simulink model "manualInputSim"  (R2025b)
settings: Solver=VariableStepAuto  StartTime=0.0  StopTime=inf  RelTol=1e-3
undefined symbols (not defined in the file or in its folder): SteerLim, VEH
libraries: sim3dlib x7, sim3dautolib x2, simulink_extras x1, vehicle_sim_lib x1
(part 1 of 2)
settings Model: Creator=bigch  LastModifiedBy=bigch

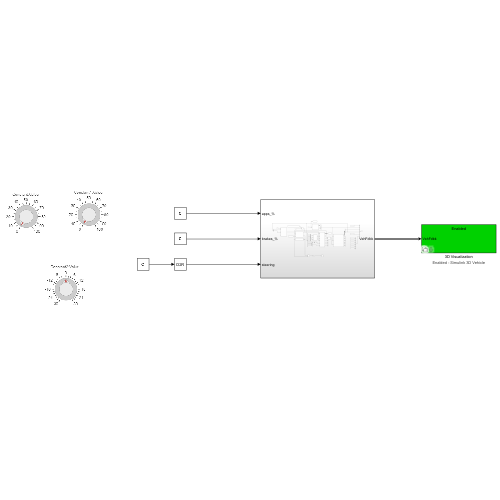
[thumbnail: Simulink's stored preview of the top-level diagram]
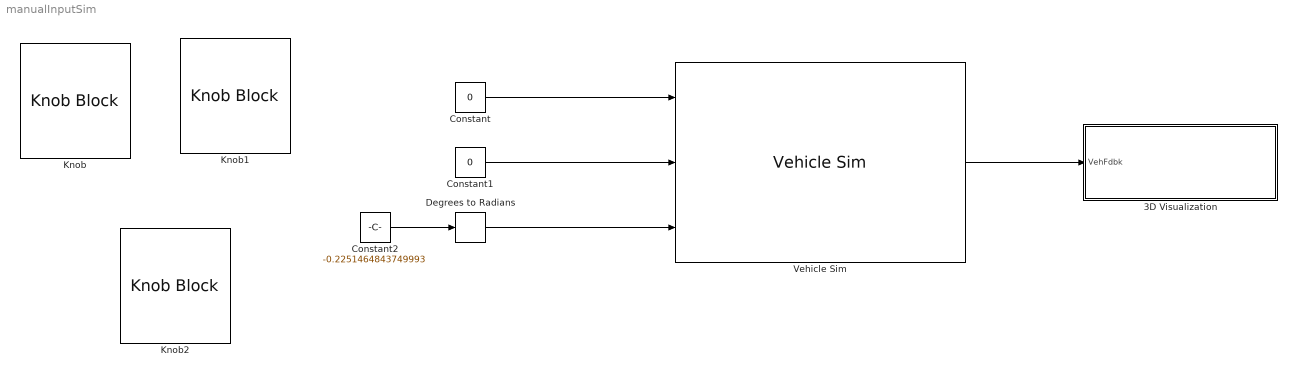
== system manualInputSim ==
  3D Visualization : Subsystem  Variant=on  VariantControl=Choice  mask(3D Visualization Setup){engine3D=Enabled - Simulink 3D Vehicle, conesOn=off, annotOn=off, pathOn=off, InitialPos=[ 0, 0, 0 ], InitialRot=[0, 0, 0], Ts=1/60}
      mask prompts: engine3D "Visualization Mode:"; conesOn "Include cones"; annotOn "Include annotations"; pathOn "Include path markers"; InitialPos "shared_sim3dblks:sim3dblkVehicleWithGroundFollowingVDBS:blkPrm_InitialPos"; InitialRot "shared_sim3dblks:sim3dblkVehicleWithGroundFollowingVDBS:blkPrm_InitialRotSAE"; Ts "shared_sim3dblks:sim3dblkConfig:Ts"
      mask help: This is an example specific block designed to only work with vydnblksskidpad.slx. It is used in conjuction with the vehicle subystem to provide options for the 3D game engine visualization (requires Simulink 3D Animation).
      mask init:
      | visType = get_param(gcb,"engine3D");
      | switch visType
      |     case "Disabled"
      |         autoblksenableparameters(gcb, [],{'conesOn';'annotOn';'pathOn'},[],[],true);
      |         set_param([bdroot '/Formula Student Vehicle'],'vehType','Simulink Physics')
      |     case "Enabled - Ground Following Vehicle"
      |         set_param([bdroot '/Formula Student Vehicle'],'vehType','Simulink Physics')
      |         autoblksenableparameters(gcb, {'conesOn';'annotOn';'pathOn'},[],[],[],true);
      |     case "Enabled - Game Physics Vehicle"
      |         set_param([bdroot '/Formula Student Vehicle'],'vehType','Game Engine Physics')
      |         autoblksenableparameters(gcb, {'conesOn';'annotOn';'pathOn'},[],[],[],true);
      | end
      settings: AttributesFormatString=%<engine3D>
      mask TypeOptions engine3D: Disabled | Enabled - Simulink 3D Vehicle | Enabled - Game Physics Vehicle
      mask Callback engine3D:
      | if strcmp(get_param(gcb,"engine3D"),"Disabled")
      |     autoblksenableparameters(gcb, [],{'conesOn';'annotOn';'pathOn'},[],[],true);
      | else
      |     autoblksenableparameters(gcb, {'conesOn';'annotOn';'pathOn'},[],[],[],true);
      | end
      mask DialogControl InitialPos Prompt: Initial position [X, Y, Z], InitialPos [m]:
      mask DialogControl InitialRot Prompt: Initial rotation [Roll, Pitch, Yaw], InitialRot [rad]:
      mask DialogControl Ts Prompt: Sample time:
  Constant : Constant  Value=0
  Constant1 : Constant  Value=0
  Constant2 : Constant  Value=-0.2251464843749993
  Degrees to Radians : simulink_extras/Transformations/Degrees to Radians
  Knob : KnobBlock
  Knob1 : KnobBlock
  Knob2 : KnobBlock  ScaleMin=-30  ScaleMax=30
  Vehicle Sim : vehicle_sim_lib/Vehicle Sim  SystemSampleTime=-1  VariantActivationTime=update diagram  EmptyChoice=off  PassThrough=off  PassThroughVariantControl=(default)  EmptyChoiceVariantControl=(default)  AllowFlexibleInterface=on  Latency=0  AutoFrameSizeCalculation=off
  wires:
  Constant1/1 -> Vehicle Sim/2
  Degrees to Radians/1 -> Vehicle Sim/3
  Vehicle Sim/1 -> 3D Visualization/1(VehFdbk)
  Constant/1 -> Vehicle Sim/1
  Constant2/1 -> Degrees to Radians/1

== system manualInputSim/3D Visualization ==
  VehFdbk : Inport
  Disabled : Subsystem  VariantControl=engine3D==1
  Enabled : Subsystem  VariantControl=engine3D~=1

== system manualInputSim/3D Visualization/Disabled ==

== system manualInputSim/3D Visualization/Enabled ==
  VehFdbk : Inport
  3D Visualization : Subsystem  Variant=on  VariantControl=Choice
  Cones : Subsystem  Variant=on  VariantControl=Choice
  wires:
  VehFdbk/1 -> 3D Visualization/1(VehFdbk)

== system manualInputSim/3D Visualization/Enabled/3D Visualization ==
  VehFdbk : Inport
  Disabled : Subsystem  VariantControl=engine3D==1
  Ground Following : Subsystem  VariantControl=engine3D==4
  Physical Vehicle : Subsystem  VariantControl=engine3D==3
  Simulation 3D Vehicle : Subsystem  VariantControl=engine3D==2

== system manualInputSim/3D Visualization/Enabled/Cones ==
  Disabled : Subsystem  VariantControl=conesOn==0
  Enabled : Subsystem  VariantControl=conesOn==1

== system manualInputSim/3D Visualization/Enabled/3D Visualization/Disabled ==

== system manualInputSim/3D Visualization/Enabled/3D Visualization/Ground Following ==
  VehFdbk : Inport
  Annotations : Subsystem  Variant=on  VariantControl=Annotations
  Bus Selector3 : BusSelector  OutputSignals=VehFdbk.InertFrm.Cg.Disp.X,VehFdbk.InertFrm.Cg.Disp.Y,VehFdbk.InertFrm.Cg.Ang.psi,Driver.Light controls
  Path : Subsystem  Variant=on  VariantControl=Choice
  Simulation 3D Scene Configuration : sim3dlib/Simulation 3D Scene Configuration  Priority=0  ProjectFormat=Default Scenes  SceneDesc=Open surface  ProjectName=C:\Program Files\MATLAB\R2025b\toolbox\shared\sim3d_projects\automotive_project_windows\UE\WindowsNoEditor\VehicleSimulation.exe  ScenePath=/Game/Maps/HwStrght  EnableOpenDRIVE=off  vehTagList={'Custom';'GamePhysVehPath';'GrndVehPath';'Scene Origin';'Sim3dActor1';'SimulinkPhysVehPath';'SimulinkVehicle1';'SimulinkVehicle2';'SimulinkVehicle3'}  vehTag=SimulinkVehicle3  AttachedCameraRelativeTranslation=[0 0 0]  FreeCameraDefaultInitialTranslation=[-6, 0, 2]  AttachedCameraRelativeRotation=[0 0 0]  FreeCameraDefaultInitialRotation=[0, -15, 0]  ViewpointName=Custom  FreeCameraInitialTranslation=[0 0 0]  ViewpointTranslation=[0 0 0]  FreeCameraInitialRotation=[0 0 0]  ViewpointRotation=[0 0 0]  OpVisEn=off  Ts=Ts  EnableWindow=on  EnableRemoteAccess=off  EnableWeather=off  SunAzimuth=90  SunAltitude=40.0  EnableGeospatialSun=off  Latitude=0  Longitude=0  Date=2023-01-01  Time=10:30:00  GeoTimeZone=-5.0  SunDaylightSaving=off  wind=1  clouds=10  EnableVolumetricClouds=off  CloudCoverage=0  CloudAltitude=6  fog=0  rain=0  RaindropsEffect=off  SnowDensity=0  EnableGeospatial=off  TilesetSource=Earth terrain  UseTrueOrigin=off  OriginHeight=200  OriginLatitude=40.744652  OriginLongitude=-73.988864  MapStyle=Aerial  AdditionalAssetIDs=[]  UseAdvancedSunSky=off  SolarTime=11  TimeZone=-5  Day=21  Month=9  Year=2022  UseDaylightSavingTime=on  DSTStartDay=10  DSTStartMonth=3  DSTEndDay=3  DSTEndMonth=11  DSTSwitchHour=2  sensorTag=MainCamera1  sensorId=1  sensorName=MainCamera1  mountLoc=Origin  offsetFlag=off  tmountOffset=[0, 0, 0]  rmountOffset=[0, 0, 0]  HorizontalResolution=1280  VerticalResolution=720  HorizontalFOV=60  mountPoint=[0 0 0]  mountOrientation=[0 0 0]  aMode=2  ID=1  GeoTrigger=Inactive  ViewNameList={'Custom'}  ViewTranslationList={'[0 0 0]'}  ViewRotationList={'[0 0 0]'}
      settings: LibrarySourceBlock=vdynlib/Vehicle Scenarios/Sim3D/Sim3D Core/Simulation 3D Scene Configuration
  Simulation 3D Vehicle with Ground Following : sim3dautolib/Simulation 3D Vehicle with Ground Following VDBS  Priority=-1  PassVehMesh=Hatchback  MeshPath=/MathWorksSimulation/Vehicles/Muscle/Meshes/SK_MuscleCar.SK_MuscleCar  TrackWidth=1.9  WheelBase=3  WheelRadius=0.35  VehColor=Red  CoordinateSystem=SAE  InitialPos=[ VEH.InitialLongPosition, VEH.InitialLatPosition, VEH.InitialVertPosition ]  InitialRot=[VEH.InitialRollAngle VEH.InitialPitchAngle VEH.InitialYawAngle]  ActorName=SimulinkVehicle3  VehLightsControl=on  HeadlightColor=[ 1, 1, 1 ]  HighBeamIntensity=100000  LowBeamIntensity=60000  HighBeamConeAngle=1.22  LowBeamConeAngle=1.22  LeftHeadlightOrientation=[ 0, 0 ]  RightHeadlightOrientation=[ 0, 0 ]  BrakelightIntensity=200  ReverselightIntensity=500  SignallightIntensity=500  SignallightPeriod=1  SignalPulseWidth=50  SampleTime=Ts  ActorType=SimulinkVehicle  ID=3  aMode=2  ActorTag=SimulinkVehicle3  CoordinateScheme=SAE
      settings: LibrarySourceBlock=vehdynlibsim3d/Simulation 3D Vehicle with Ground Following
  wires:
  Bus Selector3/1 -> Simulation 3D Vehicle with Ground Following/1  "<X>"
  VehFdbk/1 -> Path/1(VehFdbk), Annotations/1(VehFdbk), Bus Selector3/1
  Bus Selector3/2 -> Simulation 3D Vehicle with Ground Following/2  "<Y>"
  Bus Selector3/4 -> Simulation 3D Vehicle with Ground Following/4  "<Light controls>"
  Bus Selector3/3 -> Simulation 3D Vehicle with Ground Following/3  "<psi>"

== system manualInputSim/3D Visualization/Enabled/3D Visualization/Physical Vehicle ==
  VehFdbk : Inport
  Annotations : Subsystem  Variant=on  VariantControl=Annotations
  Path : Subsystem  Variant=on  VariantControl=Choice
  Simulation 3D Scene Configuration : sim3dlib/Simulation 3D Scene Configuration  Priority=0  ProjectFormat=Default Scenes  SceneDesc=Open surface  ProjectName=C:\Program Files\MATLAB\R2025b\toolbox\shared\sim3d_projects\automotive_project_windows\UE\WindowsNoEditor\VehicleSimulation.exe  ScenePath=/Game/Maps/HwStrght  UEProjPath=L:\Bsim3d\scm\automotive_project_UE4\main\src\main\AutoVrtlEnv\AutoVrtlEnv.uproject  EnableOpenDRIVE=off  vehTagList={'Custom';'GamePhysVehPath';'GrndVehPath';'Scene Origin';'Sim3dActor1';'SimulinkPhysVehPath';'SimulinkVehicle1';'SimulinkVehicle2';'SimulinkVehicle3'}  vehTag=SimulinkVehicle2  AttachedCameraRelativeTranslation=[0 0 0]  FreeCameraDefaultInitialTranslation=[-6, 0, 2]  AttachedCameraRelativeRotation=[0 0 0]  FreeCameraDefaultInitialRotation=[0, -15, 0]  ViewpointName=Custom  FreeCameraInitialTranslation=[0 0 0]  ViewpointTranslation=[0 0 0]  FreeCameraInitialRotation=[0 0 0]  ViewpointRotation=[0 0 0]  OpVisEn=off  Ts=Ts  EnableWindow=on  EnableRemoteAccess=off  EnableWeather=off  SunAzimuth=90  SunAltitude=40.0  EnableGeospatialSun=off  Latitude=0  Longitude=0  Date=2023-01-01  Time=10:30:00  GeoTimeZone=-5.0  SunDaylightSaving=off  wind=1  clouds=10  EnableVolumetricClouds=off  CloudCoverage=0  CloudAltitude=6  fog=0  rain=0  RaindropsEffect=off  SnowDensity=0  EnableGeospatial=off  TilesetSource=Earth terrain  UseTrueOrigin=off  OriginHeight=200  OriginLatitude=40.744652  OriginLongitude=-73.988864  MapStyle=Aerial  AdditionalAssetIDs=[]  UseAdvancedSunSky=off  SolarTime=11  TimeZone=-5  Day=21  Month=9  Year=2022  UseDaylightSavingTime=on  DSTStartDay=10  DSTStartMonth=3  DSTEndDay=3  DSTEndMonth=11  DSTSwitchHour=2  sensorTag=MainCamera2  sensorId=2  sensorName=MainCamera2  mountLoc=Origin  offsetFlag=off  tmountOffset=[0, 0, 0]  rmountOffset=[0, 0, 0]  HorizontalResolution=1280  VerticalResolution=720  HorizontalFOV=60  mountPoint=[0 0 0]  mountOrientation=[0 0 0]  aMode=2  ID=2  GeoTrigger=Inactive  ViewNameList={'Custom'}  ViewTranslationList={'[0 0 0]'}  ViewRotationList={'[0 0 0]'}
      settings: LibrarySourceBlock=vdynlib/Vehicle Scenarios/Sim3D/Sim3D Core/Simulation 3D Scene Configuration
  wires:
  VehFdbk/1 -> Path/1(VehFdbk), Annotations/1(VehFdbk)

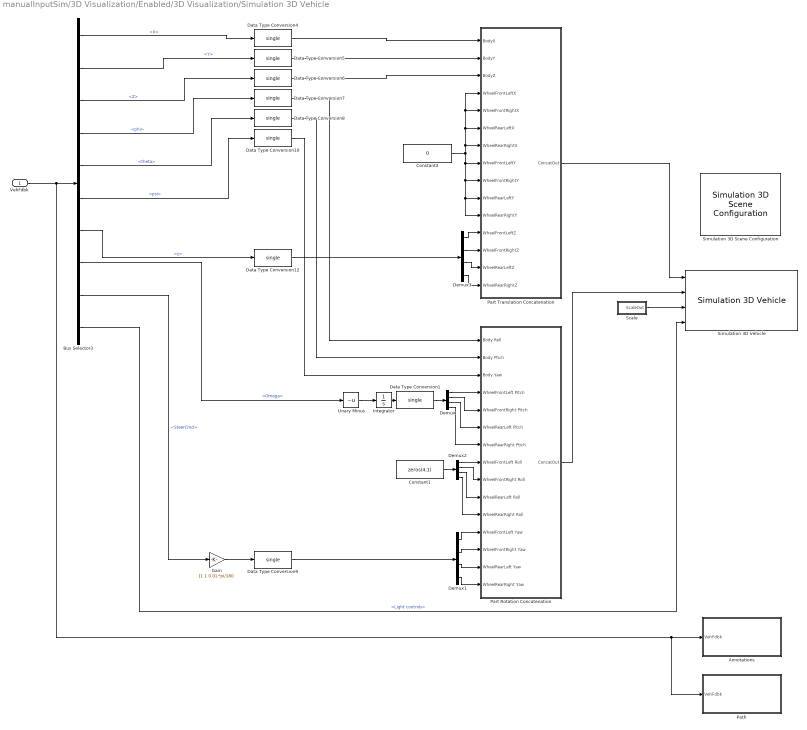
== system manualInputSim/3D Visualization/Enabled/3D Visualization/Simulation 3D Vehicle ==
  VehFdbk : Inport
  Annotations : Subsystem  Variant=on  VariantControl=Annotations
  Bus Selector3 : BusSelector  OutputSignals=InertFrm.Cg.Disp.X,InertFrm.Cg.Disp.Y,InertFrm.Cg.Disp.Z,InertFrm.Cg.Ang.phi,InertFrm.Cg.Ang.theta,InertFrm.Cg.Ang.psi,Wheels.z,Wheels.Omega,SteerCmd,Light controls
  Constant1 : Constant  Value=zeros(4,1)  OutDataTypeStr=single
  Constant2 : Constant  Value=0  OutDataTypeStr=single
  Data Type Conversion{1,4..10,12} (9 alike) : DataTypeConversion  OutDataTypeStr=single  SaturateOnIntegerOverflow=off  RndMeth=Floor
  Demux{,1..3} (4 alike) : Demux
  Gain : Gain  Gain=[1 1 0 0].*pi/180
  Integrator : Integrator  WrapState=on  WrappedStateUpperValue=2*pi  WrappedStateLowerValue=0  ZeroCross=off
  Part Rotation Concatenation : Subsystem
  Part Translation Concatenation : Subsystem
  Path : Subsystem  Variant=on  VariantControl=Choice
  Scale : Subsystem
  Simulation 3D Scene Configuration : sim3dlib/Simulation 3D Scene Configuration  Priority=0  ProjectFormat=Default Scenes  SceneDesc=Double lane change  ProjectName=C:\Program Files\MATLAB\R2025b\toolbox\shared\sim3d_projects\automotive_project_windows\UE\WindowsNoEditor\VehicleSimulation.exe  ScenePath=/Game/Maps/BlackLake  EnableOpenDRIVE=off  vehTagList={'Custom';'GamePhysVehPath';'GrndVehPath';'Scene Origin';'Sim3dActor1';'SimulinkPhysVehPath';'SimulinkVehicle1';'SimulinkVehicle3'}  vehTag=SimulinkVehicle1  AttachedCameraRelativeTranslation=[0 0 0]  FreeCameraDefaultInitialTranslation=[-6, 0, 2]  AttachedCameraRelativeRotation=[0 0 0]  FreeCameraDefaultInitialRotation=[0, -15, 0]  ViewpointName=Custom  FreeCameraInitialTranslation=[0 0 0]  ViewpointTranslation=[0 0 0]  FreeCameraInitialRotation=[0 0 0]  ViewpointRotation=[0 0 0]  OpVisEn=off  Ts=Ts  EnableWindow=on  EnableRemoteAccess=off  EnableWeather=off  SunAzimuth=90  SunAltitude=40.0  EnableGeospatialSun=off  Latitude=0  Longitude=0  Date=2023-01-01  Time=10:30:00  GeoTimeZone=-5.0  SunDaylightSaving=off  wind=1  clouds=10  EnableVolumetricClouds=off  CloudCoverage=0  CloudAltitude=6  fog=0  rain=0  RaindropsEffect=off  SnowDensity=0  EnableGeospatial=off  TilesetSource=Earth terrain  UseTrueOrigin=off  OriginHeight=200  OriginLatitude=40.744652  OriginLongitude=-73.988864  MapStyle=Aerial  AdditionalAssetIDs=[]  UseAdvancedSunSky=off  SolarTime=11  TimeZone=-5  Day=21  Month=9  Year=2022  UseDaylightSavingTime=on  DSTStartDay=10  DSTStartMonth=3  DSTEndDay=3  DSTEndMonth=11  DSTSwitchHour=2  sensorTag=MainCamera1  sensorId=1  sensorName=MainCamera1  mountLoc=Origin  offsetFlag=off  tmountOffset=[0, 0, 0]  rmountOffset=[0, 0, 0]  HorizontalResolution=1280  VerticalResolution=720  HorizontalFOV=60  mountPoint=[0 0 0]  mountOrientation=[0 0 0]  aMode=2  ID=1  GeoTrigger=Inactive  ViewNameList={'Custom'}  ViewTranslationList={'[0 0 0]'}  ViewRotationList={'[0 0 0]'}
      settings: LibrarySourceBlock=vdynlib/Vehicle Scenarios/Sim3D/Sim3D Core/Simulation 3D Scene Configuration
  Simulation 3D Vehicle : sim3dautolib/Simulation 3D Vehicle  Priority=-1  PassVehMesh=Formula student vehicle  MeshPath=/MathWorksSimulation/Vehicles/Muscle/Meshes/SK_MuscleCar.SK_MuscleCar  VehColor=Red  ActorName=SimulinkVehicle1  VehLightsControl=on  HeadlightColor=[ 1, 1, 1 ]  HighBeamIntensity=100000  LowBeamIntensity=60000  HighBeamConeAngle=1.22  LowBeamConeAngle=1.22  LeftHeadlightOrientation=[ 0, 0 ]  RightHeadlightOrientation=[ 0, 0 ]  BrakelightIntensity=500  ReverselightIntensity=500  SignallightIntensity=500  SignallightPeriod=1  SignalPulseWidth=50  Translation=[ 0, 0, 0; zeros(4,3)]  Rotation=[0 0 0; zeros( 4, 3 )]  Scale=ones( 5, 3 )  SampleTime=Ts  ActorType=SimulinkVehicle  ID=1  aMode=2  ActorTag=SimulinkVehicle1
      settings: LibrarySourceBlock=vdynlib/Vehicle Scenarios/Sim3D/Sim3D Vehicle/Components/Simulation 3D Vehicle
  Unary Minus : UnaryMinus
  wires:
  Bus Selector3/10 -> Simulation 3D Vehicle/4  "<Light controls>"
  Bus Selector3/2 -> Data Type Conversion5/1  "<Y>"
  VehFdbk/1 -> Path/1(VehFdbk), Annotations/1(VehFdbk), Bus Selector3/1
  Bus Selector3/1 -> Data Type Conversion4/1  "<X>"
  Data Type Conversion10/1 -> Part Rotation Concatenation/3(Body Yaw)
  Data Type Conversion5/1 -> Part Translation Concatenation/2(BodyY)
  Constant2/1 -> Part Translation Concatenation/4(WheelFrontLeftX), Part Translation Concatenation/5(WheelFrontRightX), Part Translation Concatenation/6(WheelRearLeftX), Part Translation Concatenation/7(WheelRearRightX), Part Translation Concatenation/8(WheelFrontLeftY), Part Translation Concatenation/9(WheelFrontRightY), Part Translation Concatenation/10(WheelRearLeftY), Part Translation Concatenation/11(WheelRearRightY)
  Data Type Conversion8/1 -> Part Rotation Concatenation/2(Body Ptich)
  Demux2/2 -> Part Rotation Concatenation/9(WheelFrontRight Roll)
  Demux1/3 -> Part Rotation Concatenation/14(WheelRearLeft Yaw)
  Demux/3 -> Part Rotation Concatenation/6(WheelRearLeft Pitch)
  Data Type Conversion9/1 -> Demux1/1
  Demux1/2 -> Part Rotation Concatenation/13(WheelFrontRight Yaw)
  Demux/2 -> Part Rotation Concatenation/5(WheelFrontRight Pitch)
  Demux2/3 -> Part Rotation Concatenation/10(WheelRearLeft Roll)
  Data Type Conversion7/1 -> Part Rotation Concatenation/1(Body Roll)
  Demux3/2 -> Part Translation Concatenation/13(WheelFrontRightZ)
  Data Type Conversion4/1 -> Part Translation Concatenation/1(BodyX)
  Integrator/1 -> Data Type Conversion1/1
  Demux2/1 -> Part Rotation Concatenation/8(WheelFrontLeft Roll)
  Demux1/4 -> Part Rotation Concatenation/15(WheelRearRight Yaw)
  Demux3/4 -> Part Translation Concatenation/15(WheelRearRightZ)
  Bus Selector3/4 -> Data Type Conversion7/1  "<phi>"
  Bus Selector3/7 -> Data Type Conversion12/1  "<z>"
  Data Type Conversion1/1 -> Demux/1
  Constant1/1 -> Demux2/1
  Demux3/3 -> Part Translation Concatenation/14(WheelRearLeftZ)
  Part Rotation Concatenation/1(ConcatOut) -> Simulation 3D Vehicle/2
  Demux3/1 -> Part Translation Concatenation/12(WheelFrontLeftZ)
  Part Translation Concatenation/1(ConcatOut) -> Simulation 3D Vehicle/1
  Demux/1 -> Part Rotation Concatenation/4(WheelFrontLeft Pitch)
  Demux1/1 -> Part Rotation Concatenation/12(WheelFrontLeft Yaw)
  Data Type Conversion6/1 -> Part Translation Concatenation/3(BodyZ)
  Unary Minus/1 -> Integrator/1
  Demux/4 -> Part Rotation Concatenation/7(WheelRearRight Ptich)
  Demux2/4 -> Part Rotation Concatenation/11(WheelRearRight Roll)
  Data Type Conversion12/1 -> Demux3/1
  Scale/1(ScaleOut) -> Simulation 3D Vehicle/3
  Bus Selector3/3 -> Data Type Conversion6/1  "<Z>"
  Bus Selector3/9 -> Gain/1  "<SteerCmd>"
  Gain/1 -> Data Type Conversion9/1
  Bus Selector3/5 -> Data Type Conversion8/1  "<theta>"
  Bus Selector3/6 -> Data Type Conversion10/1  "<psi>"
  Bus Selector3/8 -> Unary Minus/1  "<Omega>"

== system manualInputSim/3D Visualization/Enabled/Cones/Disabled ==

== system manualInputSim/3D Visualization/Enabled/Cones/Enabled ==
  Simulation 3D Actor : sim3dlib/Simulation 3D Actor  ActorName=Sim3dActor1  ParentName=Scene Origin  Operation=Create at setup  InitScriptText=|  SampleTime=Ts  Translation=single([0 0 0])  Rotation=single([0 0 0])  Scale=single([1 1 1])  aMode=5  ActorTag=Sim3dActor1  ActorType=Sim3dActor  ID=1
      | entryWidth =3.453;
      | conesZ0 = 0;
      | entryConesLoc = [entryWidth/2 -12;...
      |                  -entryWidth/2 -12;...
      |                  -entryWidth/2 -10;...
      |                  entryWidth/2 -10];
      | entryConesLoc= fliplr(entryConesLoc); % account for game engine coords
      | rightInnerRingLoc = [entryWidth/2 0;...%1
      |                   4.58/2 -2.834;...%2
      |                   7.787/2 -5.231;...%3
      |                   12.588/2 -6.835;...%4
      |                   18.25/2 -7.398;...%5
      |                   23.912/2 -6.835;...%6
      |                   28.713/2 -5.231;...%7
      |                   31.92/2 -2.834;...%8
      |                   33.047/2 0;...%9
      |                   31.92/2 2.834;...%10
      |                   28.713/2 5.231;...%11
      |                   23.912/2 6.835;...%12
      |                   18.25/2 7.398;...%13
      |                   12.588/2 6.835;...%14
      |                   7.787/2 5.231;...%15
      |                   4.58/2 2.834;...%16    
      |                   ];
      | rightInnerRingLoc = fliplr(rightInnerRingLoc);
      | leftInnerRingLoc = rightInnerRingLoc.*[1 -1];
      | rightOutterRingLoc = [entryWidth/2 7.939;...% right side entry to exit zone
      |                       9.945/2 10.026;...
      |                       18.25/2 10.852;...
      |                       26.555/2 10.026;...
      |                       33.596/2 7.673;...
      |                       38.301/2 4.153;...
      |                       39.953/2 0;...
      |                       38.301/2 -4.153;...
      |                       33.596/2 -7.673;...
      |                       26.555/2 -10.026;...
      |                       18.25/2 -10.852;...
      |                       9.945/2 -10.026;...                      
      |                       entryWidth/2 -7.939;...% right side after entry zone                      
      |                       ];
      | rightOutterRingLoc = fliplr(rightOutterRingLoc);
      | leftOutterRingLoc = rightOutterRingLoc.*[1 -1];
      | 
      | exitConesLoc = [entryWidth/2 16;...
      |                  -entryWidth/2 16;...
      |                  entryWidth/2-1 16;...
      |                  -entryWidth/2+1 16;...
      |                  -entryWidth/2 14;...
      |                  entryWidth/2 14;...
      |                  -entryWidth/2 12;...
      |                  entryWidth/2 12;...
      |                  -entryWidth/2 10;...
      |                  entryWidth/2 10];
      | exitConesLoc= fliplr(exitConesLoc); % account for game engine coords
      | 
      | timeConesLoc = fliplr([entryWidth/2 .5;...
      |                  -entryWidth/2 .5;...
      |                  entryWidth/2 -.5;...
      |                  -entryWidth/2 -.5]);
      | 
      | blueCones = [rightOutterRingLoc; leftInnerRingLoc];
      | yellowCones = [rightInnerRingLoc; leftOutterRingLoc];
      | smallOrangeCones = [entryConesLoc; exitConesLoc];
      | largeOrangeCones = timeConesLoc;
      | 
      | skidSurface = sim3d.Actor('ActorName','BaseSurface');
      | skidSurface.createShape('box',[45,45,+0.03]);
      | skidSurface.Color = [68 68 71]./100;
      | skidSurface.Translation = [0 0 0]; 
      | skidSurface.Texture = fullfile(pwd,"vdynskidpad.png"); 
      | skidSurface.TextureTransform.Scale = [1 1];
      | skidSurface.TextureTransform.Angle = 0;
      | skidSurface.Shininess = 0;
      | skidSurface.Transparency = 0;
      | skidSurface.TextureMapping.Blend = 1;
      | skidSurface.TextureMapping.Roughness = .8;
      | World.add(skidSurface,Actor);
      | 
      | nCones = length(largeOrangeCones);
      | for coneNum = 1:nCones    
      |     coneName = "LCone_" + num2str(coneNum);
      |     conLoc = [largeOrangeCones(coneNum,:) conesZ0];
      |     cone = sim3d.Actor('ActorName',coneName,'Mesh','/Game/Environment/Industrial/Props/Cone/Mesh/SM_Cone.SM_Cone',...
      |         'Mobility', sim3d.utils.MobilityTypes.Movable,...
      |         'SimulatePhysics', true,...
      |         'Translation',conLoc,...
      |         'EnableGravity', true);    
      |     %cone.Shadows = true;
      |     World.add(cone,Actor);
      | end
      | 
      | %smallCones = [blueCones; yellowCones; smallOrangeCones]; 
      | 
      | 
      | for coneNum = 1:length(blueCones)    
      |     coneName = "bCone_" + num2str(coneNum);
      |     conLoc = [blueCones(coneNum,:) conesZ0];
      |     cone = sim3d.Actor('ActorName',coneName,'Mesh','/Game/Environment/Industrial/Props/Cone/Mesh/SM_Cone_Blue.SM_Cone_Blue',...
      |         'Mobility', sim3d.utils.MobilityTypes.Movable,...
      |         'SimulatePhysics', true,...
      |         'Translation',conLoc,...
      |         'EnableGravity', true,...
      |         'Scale',ones(1,3).*325/500);    
      |     %cone.Color= [102 140 204]./255;
      |     World.add(cone,Actor);
      | end
      | for coneNum = 1:length(yellowCones)    
      |     coneName = "yCone_" + num2str(coneNum);
      |     conLoc = [yellowCones(coneNum,:) conesZ0];
      |     cone = sim3d.Actor('ActorName',coneName,'Mesh','/Game/Environment/Industrial/Props/Cone/Mesh/SM_Cone_Yellow.SM_Cone_Yellow',...
      |         'Mobility', sim3d.utils.MobilityTypes.Movable,...
      |         'SimulatePhysics', true,...
      |         'Translation',conLoc,...
      |         'EnableGravity', true,...
      |         'Scale',ones(1,3).*325/500);    
      |     %cone.Color= [102 140 204]./255;
      |     World.add(cone,Actor);
      | end
      | for coneNum = 1:length(smallOrangeCones)    
      |     coneName = "sCone_" + num2str(coneNum);
      |     conLoc = [smallOrangeCones(coneNum,:) conesZ0];
      |     cone = sim3d.Actor('ActorName',coneName,'Mesh','/Game/Environment/Industrial/Props/Cone/Mesh/SM_Cone.SM_Cone',...
      |         'Mobility', sim3d.utils.MobilityTypes.Movable,...
      |         'SimulatePhysics', true,...
      |         'Translation',conLoc,...
      |         'EnableGravity', true,...
      |         'Scale',ones(1,3).*325/500);    
      |     %cone.Color= [102 140 204]./255;
      |     World.add(cone,Actor);
      | end
      settings: LibrarySourceBlock=sl3dlib/Simulation 3D/Simulation 3D Actor
  Terminator : Terminator
  wires:
  Simulation 3D Actor/1 -> Terminator/1

== system manualInputSim/3D Visualization/Enabled/3D Visualization/Ground Following/Annotations ==
  VehFdbk : Inport
  Disabled : Subsystem  VariantControl=annotOn==0
  Enabled : Subsystem  VariantControl=annotOn==1

== system manualInputSim/3D Visualization/Enabled/3D Visualization/Ground Following/Path ==
  VehFdbk : Inport
  Disabled : Subsystem  VariantControl=pathOn==0
  Enabled : Subsystem  VariantControl=pathOn==1

== system manualInputSim/3D Visualization/Enabled/3D Visualization/Physical Vehicle/Annotations ==
  VehFdbk : Inport
  Disabled : Subsystem  VariantControl=annotOn==0
  Enabled : Subsystem  VariantControl=annotOn==1

== system manualInputSim/3D Visualization/Enabled/3D Visualization/Physical Vehicle/Path ==
  VehFdbk : Inport
  Disabled : Subsystem  VariantControl=pathOn==0
  Enabled : Subsystem  VariantControl=pathOn==1

== system manualInputSim/3D Visualization/Enabled/3D Visualization/Simulation 3D Vehicle/Annotations ==
  VehFdbk : Inport
  Disabled : Subsystem  VariantControl=annotOn==0
  Enabled : Subsystem  VariantControl=annotOn==1

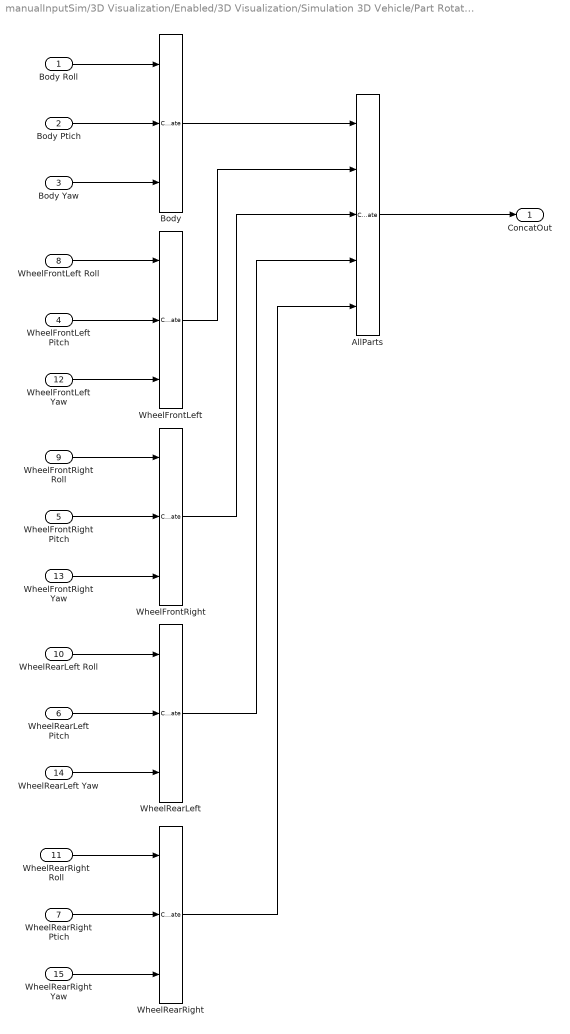
== system manualInputSim/3D Visualization/Enabled/3D Visualization/Simulation 3D Vehicle/Part Rotation Concatenation ==
  Body Roll : Inport
  Body Ptich : Inport  Port=2
  Body Yaw : Inport  Port=3
  WheelFrontLeft Pitch : Inport  Port=4
  WheelFrontRight Pitch : Inport  Port=5
  WheelRearLeft Pitch : Inport  Port=6
  WheelRearRight Ptich : Inport  Port=7
  WheelFrontLeft Roll : Inport  Port=8
  WheelFrontRight Roll : Inport  Port=9
  WheelRearLeft Roll : Inport  Port=10
  WheelRearRight Roll : Inport  Port=11
  WheelFrontLeft Yaw : Inport  Port=12
  WheelFrontRight Yaw : Inport  Port=13
  WheelRearLeft Yaw : Inport  Port=14
  WheelRearRight Yaw : Inport  Port=15
  AllParts : Concatenate  NumInputs=5  Mode=Multidimensional array
  Body : Concatenate  NumInputs=3  Mode=Multidimensional array  ConcatenateDimension=2
  WheelFrontLeft : Concatenate  NumInputs=3  Mode=Multidimensional array  ConcatenateDimension=2
  WheelFrontRight : Concatenate  NumInputs=3  Mode=Multidimensional array  ConcatenateDimension=2
  WheelRearLeft : Concatenate  NumInputs=3  Mode=Multidimensional array  ConcatenateDimension=2
  WheelRearRight : Concatenate  NumInputs=3  Mode=Multidimensional array  ConcatenateDimension=2
  ConcatOut : Outport  VectorParamsAs1DForOutWhenUnconnected=off
  wires:
  Body Yaw/1 -> Body/3
  WheelFrontLeft Yaw/1 -> WheelFrontLeft/3
  WheelFrontLeft/1 -> AllParts/2
  Body/1 -> AllParts/1
  WheelRearLeft/1 -> AllParts/4
  WheelFrontRight/1 -> AllParts/3
  WheelRearRight Yaw/1 -> WheelRearRight/3
  WheelRearLeft Yaw/1 -> WheelRearLeft/3
  AllParts/1 -> ConcatOut/1
  WheelRearRight/1 -> AllParts/5
  WheelFrontRight Yaw/1 -> WheelFrontRight/3
  Body Ptich/1 -> Body/2
  Body Roll/1 -> Body/1
  WheelFrontLeft Pitch/1 -> WheelFrontLeft/2
  WheelFrontLeft Roll/1 -> WheelFrontLeft/1
  WheelFrontRight Pitch/1 -> WheelFrontRight/2
  WheelFrontRight Roll/1 -> WheelFrontRight/1
  WheelRearLeft Pitch/1 -> WheelRearLeft/2
  WheelRearLeft Roll/1 -> WheelRearLeft/1
  WheelRearRight Ptich/1 -> WheelRearRight/2
  WheelRearRight Roll/1 -> WheelRearRight/1

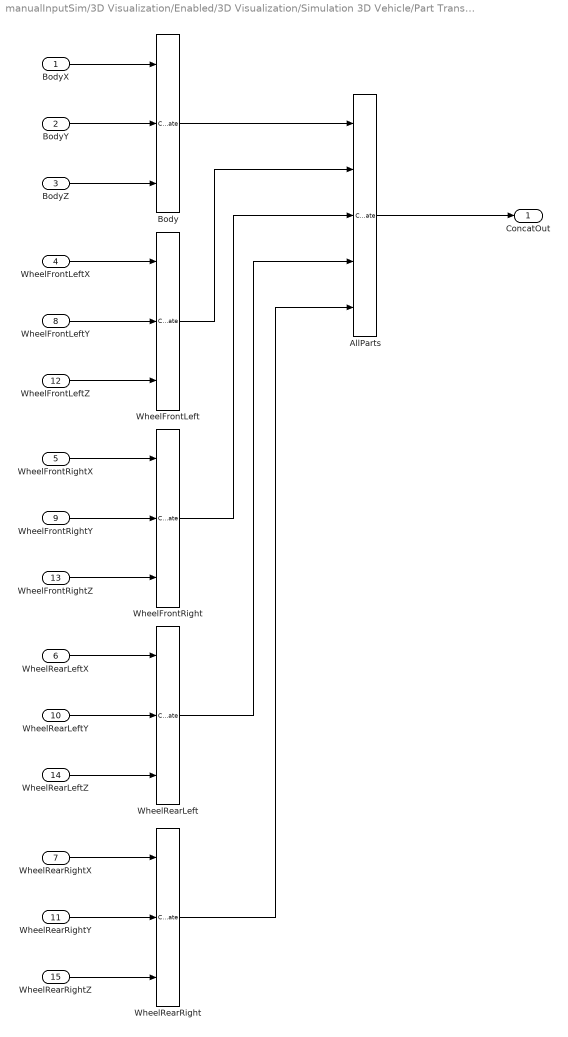
== system manualInputSim/3D Visualization/Enabled/3D Visualization/Simulation 3D Vehicle/Part Translation Concatenation ==
  BodyX : Inport
  BodyY : Inport  Port=2
  BodyZ : Inport  Port=3
  WheelFrontLeftX : Inport  Port=4
  WheelFrontRightX : Inport  Port=5
  WheelRearLeftX : Inport  Port=6
  WheelRearRightX : Inport  Port=7
  WheelFrontLeftY : Inport  Port=8
  WheelFrontRightY : Inport  Port=9
  WheelRearLeftY : Inport  Port=10
  WheelRearRightY : Inport  Port=11
  WheelFrontLeftZ : Inport  Port=12
  WheelFrontRightZ : Inport  Port=13
  WheelRearLeftZ : Inport  Port=14
  WheelRearRightZ : Inport  Port=15
  AllParts : Concatenate  NumInputs=5  Mode=Multidimensional array
  Body : Concatenate  NumInputs=3  Mode=Multidimensional array  ConcatenateDimension=2
  WheelFrontLeft : Concatenate  NumInputs=3  Mode=Multidimensional array  ConcatenateDimension=2
  WheelFrontRight : Concatenate  NumInputs=3  Mode=Multidimensional array  ConcatenateDimension=2
  WheelRearLeft : Concatenate  NumInputs=3  Mode=Multidimensional array  ConcatenateDimension=2
  WheelRearRight : Concatenate  NumInputs=3  Mode=Multidimensional array  ConcatenateDimension=2
  ConcatOut : Outport  VectorParamsAs1DForOutWhenUnconnected=off
  wires:
  BodyX/1 -> Body/1
  BodyZ/1 -> Body/3
  WheelFrontLeftX/1 -> WheelFrontLeft/1
  WheelFrontLeftZ/1 -> WheelFrontLeft/3
  WheelFrontLeftY/1 -> WheelFrontLeft/2
  BodyY/1 -> Body/2
  WheelFrontLeft/1 -> AllParts/2
  WheelRearRightX/1 -> WheelRearRight/1
  Body/1 -> AllParts/1
  WheelRearLeft/1 -> AllParts/4
  WheelFrontRight/1 -> AllParts/3
  WheelRearRightZ/1 -> WheelRearRight/3
  WheelFrontRightY/1 -> WheelFrontRight/2
  WheelFrontRightX/1 -> WheelFrontRight/1
  WheelRearRightY/1 -> WheelRearRight/2
  WheelRearLeftZ/1 -> WheelRearLeft/3
  AllParts/1 -> ConcatOut/1
  WheelRearLeftY/1 -> WheelRearLeft/2
  WheelRearRight/1 -> AllParts/5
  WheelRearLeftX/1 -> WheelRearLeft/1
  WheelFrontRightZ/1 -> WheelFrontRight/3

== system manualInputSim/3D Visualization/Enabled/3D Visualization/Simulation 3D Vehicle/Path ==
  VehFdbk : Inport
  Disabled : Subsystem  VariantControl=pathOn==0
  Enabled : Subsystem  VariantControl=pathOn==1

== system manualInputSim/3D Visualization/Enabled/3D Visualization/Simulation 3D Vehicle/Scale ==
  Constant{1..12,17,32..33} (15 alike) : Constant  OutDataTypeStr=single
  PartConcatenation : Subsystem
  ScaleOut : Outport  VectorParamsAs1DForOutWhenUnconnected=off
  wires:
  Constant10/1 -> PartConcatenation/15(WheelRearRightZ)
  Constant9/1 -> PartConcatenation/14(WheelRearRightY)
  Constant11/1 -> PartConcatenation/13(WheelRearRightX)
  Constant7/1 -> PartConcatenation/12(WheelRearLeftZ)
  Constant6/1 -> PartConcatenation/11(WheelRearLeftY)
  Constant8/1 -> PartConcatenation/10(WheelRearLeftX)
  Constant4/1 -> PartConcatenation/9(WheelFrontRightZ)
  Constant3/1 -> PartConcatenation/8(WheelFrontRightY)
  Constant5/1 -> PartConcatenation/7(WheelFrontRightX)
  Constant2/1 -> PartConcatenation/6(WheelFrontLeftZ)
  Constant1/1 -> PartConcatenation/5(WheelFrontLeftY)
  Constant33/1 -> PartConcatenation/4(WheelFrontLeftX)
  Constant32/1 -> PartConcatenation/3(BodyZ)
  Constant17/1 -> PartConcatenation/2(BodyY)
  Constant12/1 -> PartConcatenation/1(BodyX)
  PartConcatenation/1(ConcatOut) -> ScaleOut/1

== system manualInputSim/3D Visualization/Enabled/3D Visualization/Ground Following/Annotations/Disabled ==

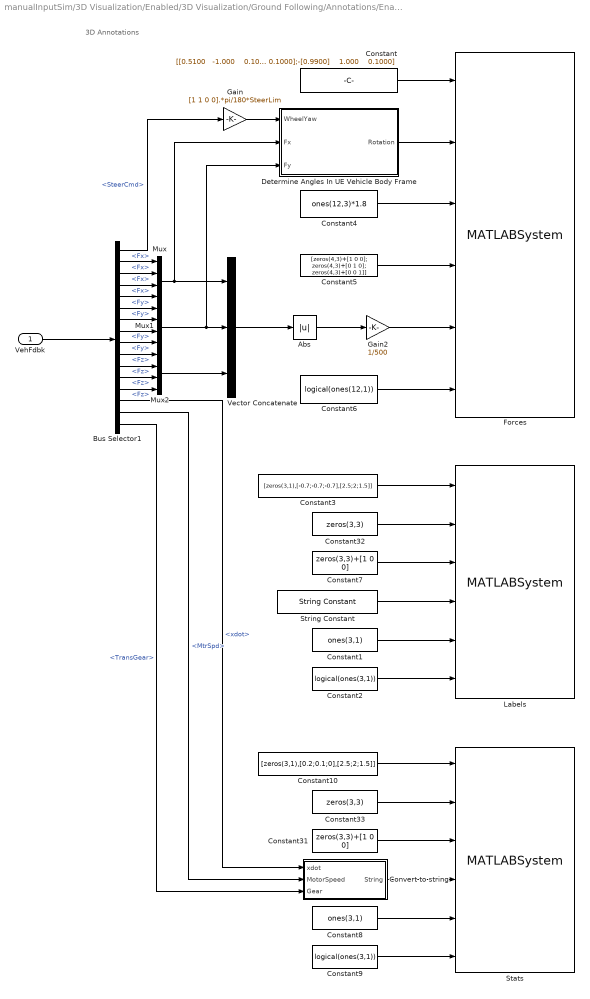
== system manualInputSim/3D Visualization/Enabled/3D Visualization/Ground Following/Annotations/Enabled ==
  note: 3D Annotations
  VehFdbk : Inport
  Abs : Abs  ZeroCross=off  SaturateOnIntegerOverflow=off
  Bus Selector1 : BusSelector  OutputSignals=Driver.SteerCmd,VehFdbk.BdyFrm.Forces.Tires.FrntTires.Lft.Fx,VehFdbk.BdyFrm.Forces.Tires.FrntTires.Rght.Fx,VehFdbk.BdyFrm.Forces.Tires.RearTires.Lft.Fx,VehFdbk.BdyFrm.Forces.Tires.RearTires.Rght.Fx,VehFdbk.BdyFrm.Forces.Tires.FrntTires.Lft.Fy,VehFdbk.BdyFrm.Forces.Tires.FrntTires.Rght.Fy,VehFdbk.BdyFrm.Forces.Tires.RearTires.Lft.Fy,VehFdbk.BdyFrm.Forces.Tires.RearTires.Rght.Fy,VehFdbk.BdyFrm.Forces.Tires.FrntTires.Lft.Fz,VehFdbk.BdyFrm.Forces.Tires.FrntTires.Rght.Fz,VehFdbk.BdyFrm.Forces.Tires.RearTires.Lft.Fz,VehFdbk.BdyFrm.Forces.Tires.RearTires.Rght.Fz,VehFdbk.BdyFrm.Cg.Vel.xdot,VehFdbk.Mtr.MtrSpd,VehFdbk.Trans.TransGear
  Constant : Constant  Value="[[0.5100   -1.000    0.1000];[0.5100    1.000    0.1000];[-0.9900   -1.000    0.1000];[-0.9900    1.000    0.1000];[0.5100   -1.000    0.1000];[0.5100    1.000    0.1000];[-0.9900   -1.000    0.1000];[-0.9900    1.000    0.1000];[0.5100   -1.000    0.1000];[0.5100    1.000    0.1000];[-0.9900   -1.000    0.1000];-[0.9900]    1.000    0.1000]"
  Constant1 : Constant  Value=ones(3,1)
  Constant10 : Constant  Value=[zeros(3,1),[0.2;0.1;0],[2.5;2;1.5]]
  Constant2 : Constant  Value=logical(ones(3,1))
  Constant3 : Constant  Value=[zeros(3,1),[-0.7;-0.7;-0.7],[2.5;2;1.5]]
  Constant31 : Constant  Value=zeros(3,3)+[1 0 0]
  Constant32 : Constant  Value=zeros(3,3)
  Constant33 : Constant  Value=zeros(3,3)
  Constant4 : Constant  Value=ones(12,3)*1.8
  Constant5 : Constant  Value=[zeros(4,3)+[1 0 0]; zeros(4,3)+[0 1 0]; zeros(4,3)+[0 0 1]]
  Constant6 : Constant  Value=logical(ones(12,1))
  Constant7 : Constant  Value=zeros(3,3)+[1 0 0]
  Constant8 : Constant  Value=ones(3,1)
  Constant9 : Constant  Value=logical(ones(3,1))
  Convert to string : Subsystem
  Determine Angles In UE Vehicle Body Frame : Subsystem
  Forces : MATLABSystem  Priority=-1  System=Simulation3DAnnotation  InitialPos="[[0.5100   -1.000    0.1000];[0.5100    1.000    0.1000];[-0.9900   -1.000    0.1000];[-0.9900    1.000    0.1000];[0.5100   -1.000    0.1000];[0.5100    1.000    0.1000];[-0.9900   -1.000    0.1000];[-0.9900    1.000    0.1000];[0.5100   -1.000    0.1000];[0.5100    1.000    0.1000];[-0.9900   -1.000    0.1000];-[0.9900]    1.000    0.1000]"  InitialRot=[zeros(4,3);[zeros(4,3)+[0 0 pi/2]];[zeros(4,3)+[0 pi/2 0]]]  InitialScale=zeros(12,3)  ActorTag=AnnotationActor1  ParentActor=SimulinkVehicle2  Color=[zeros(4,3)+[1 0 0]; zeros(4,3)+[0 1 0]; zeros(4,3)+[0 0 1]]  Length=zeros(12,1)  FontScale=1  IsHidden=logical(zeros(12,1))  SampleTime=Ts
      mask Type: Simulation3DAnnotation
  Gain : Gain  Gain=[1 1 0 0].*pi/180*SteerLim
  Gain2 : Gain  Gain=1/500
  Labels : MATLABSystem  Priority=-1  System=Simulation3DAnnotation  InitialPos=[zeros(3,1),[-0.7;-0.7;-0.7],[2.5;2;1.5]]  InitialRot=zeros(3,3)  InitialScale=zeros(3,3)  ActorTag=AnnotationActor2  ParentActor=SimulinkVehicle2  Color=zeros(3,3)+[1 0 0]  Length=1  String=Velocity\n Engine\n Gear  FontScale=ones(3,1)  IsHidden=logical(ones(3,1))  SampleTime=Ts
      mask Type: Simulation3DAnnotation
  Mux : Mux
  Mux1 : Mux
  Mux2 : Mux
  Stats : MATLABSystem  Priority=-1  System=Simulation3DAnnotation  InitialPos=[zeros(3,1),[0.2;0.1;0],[2.5;2;1.5]]  InitialRot=zeros(3,3)  InitialScale=zeros(3,3)  ActorTag=AnnotationActor3  ParentActor=SimulinkVehicle2  Color=zeros(3,3)+[1 0 0]  Length=1  String=00 km/h\n 0000 RPM\n 0  FontScale=ones(3,1)  IsHidden=logical(ones(3,1))  SampleTime=Ts
      mask Type: Simulation3DAnnotation
  String Constant : StringConstant  String="\"Velocity\\n Engine\\n Gear\""
  Vector Concatenate : Concatenate  NumInputs=3
  wires:
  VehFdbk/1 -> Bus Selector1/1
  Determine Angles In UE Vehicle Body Frame/1(Rotation) -> Forces/2
  Mux/1 -> Vector Concatenate/1, Determine Angles In UE Vehicle Body Frame/2(Fx)
  Mux1/1 -> Determine Angles In UE Vehicle Body Frame/3(Fy), Vector Concatenate/2
  Bus Selector1/1 -> Gain/1  "<SteerCmd>"
  Convert to string/1(String) -> Stats/4
  String Constant/1 -> Labels/4
  Constant33/1 -> Stats/2
  Constant31/1 -> Stats/3
  Constant8/1 -> Stats/5
  Constant9/1 -> Stats/6
  Constant32/1 -> Labels/2
  Constant3/1 -> Labels/1
  Constant7/1 -> Labels/3
  Constant1/1 -> Labels/5
  Constant2/1 -> Labels/6
  Constant10/1 -> Stats/1
  Constant/1 -> Forces/1
  Mux2/1 -> Vector Concatenate/3
  Abs/1 -> Gain2/1
  Vector Concatenate/1 -> Abs/1
  Gain2/1 -> Forces/5
  Constant4/1 -> Forces/3
  Constant6/1 -> Forces/6
  Constant5/1 -> Forces/4
  Gain/1 -> Determine Angles In UE Vehicle Body Frame/1(WheelYaw)
  Bus Selector1/2 -> Mux/1  "<Fx>"
  Bus Selector1/3 -> Mux/2  "<Fx>"
  Bus Selector1/4 -> Mux/3  "<Fx>"
  Bus Selector1/5 -> Mux/4  "<Fx>"
  Bus Selector1/6 -> Mux1/1  "<Fy>"
  Bus Selector1/7 -> Mux1/2  "<Fy>"
  Bus Selector1/8 -> Mux1/3  "<Fy>"
  Bus Selector1/9 -> Mux1/4  "<Fy>"
  Bus Selector1/10 -> Mux2/1  "<Fz>"
  Bus Selector1/11 -> Mux2/2  "<Fz>"
  Bus Selector1/12 -> Mux2/3  "<Fz>"
  Bus Selector1/13 -> Mux2/4  "<Fz>"
  Bus Selector1/14 -> Convert to string/1(xdot)  "<xdot>"
  Bus Selector1/15 -> Convert to string/2(MotorSpeed)  "<MtrSpd>"
  Bus Selector1/16 -> Convert to string/3(Gear)  "<TransGear>"

== system manualInputSim/3D Visualization/Enabled/3D Visualization/Ground Following/Path/Disabled ==

== system manualInputSim/3D Visualization/Enabled/3D Visualization/Ground Following/Path/Enabled ==
  VehFdbk : Inport
  Bus Selector : BusSelector  OutputSignals=VehFdbk.BdyFrm.Cg.Acc.ax,VehFdbk.BdyFrm.Cg.Acc.ay
  Constant5 : Constant
  Constant6 : Constant  Value=0
  Hypot : Math  Operator=hypot
  Saturation : Saturate  UpperLimit=1  LowerLimit=0  ZeroCross=off
  Simulation 3D Actor : sim3dlib/Simulation 3D Actor  ActorName=GrndVehPath  ParentName=Scene Origin  Operation=Create at setup  InitScriptText=|  SampleTime=Ts*5  Translation=[0 0 0]  Rotation=[0 0 0]  Scale=[1 1 1]  InputsText=PathMarker.Color  aMode=5  ActorTag=GrndVehPath  ActorType=Sim3dActor  ID=C
      | path1 = sim3d.graphics.PathMarker("ActorName", "PathMarker", ControlActorName="SimulinkVehicle3");
      | path1.MarkersSize = ones(1,3)*0.25;
      | path1.Color = [0 0 1];
      | World.add(path1,Actor);
  Sum1 : Sum  Inputs=|++
  Terminator4 : Terminator
  Unary Minus : UnaryMinus
  Vector Concatenate : Concatenate  NumInputs=3  Mode=Multidimensional array  ConcatenateDimension=2
  wires:
  Hypot/1 -> Saturation/1
  Saturation/1 -> Unary Minus/1, Vector Concatenate/1
  Constant5/1 -> Sum1/2
  Simulation 3D Actor/1 -> Terminator4/1
  Sum1/1 -> Vector Concatenate/3
  Unary Minus/1 -> Sum1/1
  Constant6/1 -> Vector Concatenate/2
  VehFdbk/1 -> Bus Selector/1
  Bus Selector/2 -> Hypot/2  "<ay>"
  Bus Selector/1 -> Hypot/1  "<ax>"
  Vector Concatenate/1 -> Simulation 3D Actor/1

== system manualInputSim/3D Visualization/Enabled/3D Visualization/Physical Vehicle/Annotations/Disabled ==

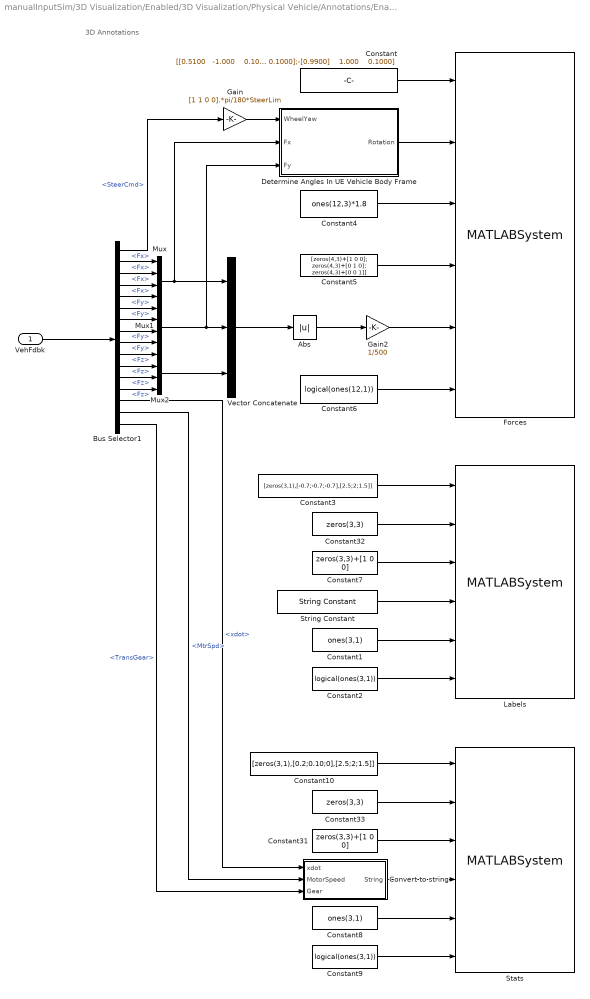
== system manualInputSim/3D Visualization/Enabled/3D Visualization/Physical Vehicle/Annotations/Enabled ==
  note: 3D Annotations
  VehFdbk : Inport
  Abs : Abs  ZeroCross=off  SaturateOnIntegerOverflow=off
  Bus Selector1 : BusSelector  OutputSignals=Driver.SteerCmd,VehFdbk.BdyFrm.Forces.Tires.FrntTires.Lft.Fx,VehFdbk.BdyFrm.Forces.Tires.FrntTires.Rght.Fx,VehFdbk.BdyFrm.Forces.Tires.RearTires.Lft.Fx,VehFdbk.BdyFrm.Forces.Tires.RearTires.Rght.Fx,VehFdbk.BdyFrm.Forces.Tires.FrntTires.Lft.Fy,VehFdbk.BdyFrm.Forces.Tires.FrntTires.Rght.Fy,VehFdbk.BdyFrm.Forces.Tires.RearTires.Lft.Fy,VehFdbk.BdyFrm.Forces.Tires.RearTires.Rght.Fy,VehFdbk.BdyFrm.Forces.Tires.FrntTires.Lft.Fz,VehFdbk.BdyFrm.Forces.Tires.FrntTires.Rght.Fz,VehFdbk.BdyFrm.Forces.Tires.RearTires.Lft.Fz,VehFdbk.BdyFrm.Forces.Tires.RearTires.Rght.Fz,VehFdbk.BdyFrm.Cg.Vel.xdot,VehFdbk.Mtr.MtrSpd,VehFdbk.Trans.TransGear
  Constant : Constant  Value="[[0.5100   -1.000    0.1000];[0.5100    1.000    0.1000];[-0.9900   -1.000    0.1000];[-0.9900    1.000    0.1000];[0.5100   -1.000    0.1000];[0.5100    1.000    0.1000];[-0.9900   -1.000    0.1000];[-0.9900    1.000    0.1000];[0.5100   -1.000    0.1000];[0.5100    1.000    0.1000];[-0.9900   -1.000    0.1000];-[0.9900]    1.000    0.1000]"
  Constant1 : Constant  Value=ones(3,1)
  Constant10 : Constant  Value=[zeros(3,1),[0.2;0.10;0],[2.5;2;1.5]]
  Constant2 : Constant  Value=logical(ones(3,1))
  Constant3 : Constant  Value=[zeros(3,1),[-0.7;-0.7;-0.7],[2.5;2;1.5]]
  Constant31 : Constant  Value=zeros(3,3)+[1 0 0]
  Constant32 : Constant  Value=zeros(3,3)
  Constant33 : Constant  Value=zeros(3,3)
  Constant4 : Constant  Value=ones(12,3)*1.8
  Constant5 : Constant  Value=[zeros(4,3)+[1 0 0]; zeros(4,3)+[0 1 0]; zeros(4,3)+[0 0 1]]
  Constant6 : Constant  Value=logical(ones(12,1))
  Constant7 : Constant  Value=zeros(3,3)+[1 0 0]
  Constant8 : Constant  Value=ones(3,1)
  Constant9 : Constant  Value=logical(ones(3,1))
  Convert to string : Subsystem
  Determine Angles In UE Vehicle Body Frame : Subsystem
  Forces : MATLABSystem  Priority=-1  System=Simulation3DAnnotation  InitialPos="[[0.5100   -1.000    0.1000];[0.5100    1.000    0.1000];[-0.9900   -1.000    0.1000];[-0.9900    1.000    0.1000];[0.5100   -1.000    0.1000];[0.5100    1.000    0.1000];[-0.9900   -1.000    0.1000];[-0.9900    1.000    0.1000];[0.5100   -1.000    0.1000];[0.5100    1.000    0.1000];[-0.9900   -1.000    0.1000];-[0.9900]    1.000    0.1000]"  InitialRot=[zeros(4,3);[zeros(4,3)+[0 0 pi/2]];[zeros(4,3)+[0 pi/2 0]]]  InitialScale=zeros(12,3)  ActorTag=AnnotationActor1  ParentActor=SimulinkVehicle2  Color=[zeros(4,3)+[1 0 0]; zeros(4,3)+[0 1 0]; zeros(4,3)+[0 0 1]]  Length=zeros(12,1)  FontScale=1  IsHidden=logical(zeros(12,1))  SampleTime=Ts
      mask Type: Simulation3DAnnotation
  Gain : Gain  Gain=[1 1 0 0].*pi/180*SteerLim
  Gain2 : Gain  Gain=1/500
  Labels : MATLABSystem  Priority=-1  System=Simulation3DAnnotation  InitialPos=[zeros(3,1),[-0.7;-0.7;-0.7],[2.5;2;1.5]]  InitialRot=zeros(3,3)  InitialScale=zeros(3,3)  ActorTag=AnnotationActor2  ParentActor=SimulinkVehicle2  Color=zeros(3,3)+[1 0 0]  Length=1  String=Velocity\n Engine\n Gear  FontScale=ones(3,1)  IsHidden=logical(ones(3,1))  SampleTime=Ts
      mask Type: Simulation3DAnnotation
  Mux : Mux
  Mux1 : Mux
  Mux2 : Mux
  Stats : MATLABSystem  Priority=-1  System=Simulation3DAnnotation  InitialPos=[zeros(3,1),[0.2;0.1;0.0],[2.5;2;1.5]]  InitialRot=zeros(3,3)  InitialScale=zeros(3,3)  ActorTag=AnnotationActor3  ParentActor=SimulinkVehicle2  Color=zeros(3,3)+[1 0 0]  Length=1  String=00 km/h\n 0000 RPM\n 0  FontScale=ones(3,1)  IsHidden=logical(ones(3,1))  SampleTime=Ts
      mask Type: Simulation3DAnnotation
  String Constant : StringConstant  String="\"Velocity\\n Engine\\n Gear\""
  Vector Concatenate : Concatenate  NumInputs=3
  wires:
  VehFdbk/1 -> Bus Selector1/1
  Determine Angles In UE Vehicle Body Frame/1(Rotation) -> Forces/2
  Mux/1 -> Vector Concatenate/1, Determine Angles In UE Vehicle Body Frame/2(Fx)
  Mux1/1 -> Determine Angles In UE Vehicle Body Frame/3(Fy), Vector Concatenate/2
  Bus Selector1/1 -> Gain/1  "<SteerCmd>"
  Convert to string/1(String) -> Stats/4
  String Constant/1 -> Labels/4
  Constant33/1 -> Stats/2
  Constant31/1 -> Stats/3
  Constant8/1 -> Stats/5
  Constant9/1 -> Stats/6
  Constant32/1 -> Labels/2
  Constant3/1 -> Labels/1
  Constant7/1 -> Labels/3
  Constant1/1 -> Labels/5
  Constant2/1 -> Labels/6
  Constant10/1 -> Stats/1
  Constant/1 -> Forces/1
  Mux2/1 -> Vector Concatenate/3
  Abs/1 -> Gain2/1
  Vector Concatenate/1 -> Abs/1
  Gain2/1 -> Forces/5
  Constant4/1 -> Forces/3
  Constant6/1 -> Forces/6
  Constant5/1 -> Forces/4
  Gain/1 -> Determine Angles In UE Vehicle Body Frame/1(WheelYaw)
  Bus Selector1/2 -> Mux/1  "<Fx>"
  Bus Selector1/3 -> Mux/2  "<Fx>"
  Bus Selector1/4 -> Mux/3  "<Fx>"
  Bus Selector1/5 -> Mux/4  "<Fx>"
  Bus Selector1/6 -> Mux1/1  "<Fy>"
  Bus Selector1/7 -> Mux1/2  "<Fy>"
  Bus Selector1/8 -> Mux1/3  "<Fy>"
  Bus Selector1/9 -> Mux1/4  "<Fy>"
  Bus Selector1/10 -> Mux2/1  "<Fz>"
  Bus Selector1/11 -> Mux2/2  "<Fz>"
  Bus Selector1/12 -> Mux2/3  "<Fz>"
  Bus Selector1/13 -> Mux2/4  "<Fz>"
  Bus Selector1/14 -> Convert to string/1(xdot)  "<xdot>"
  Bus Selector1/15 -> Convert to string/2(MotorSpeed)  "<MtrSpd>"
  Bus Selector1/16 -> Convert to string/3(Gear)  "<TransGear>"

== system manualInputSim/3D Visualization/Enabled/3D Visualization/Physical Vehicle/Path/Disabled ==

== system manualInputSim/3D Visualization/Enabled/3D Visualization/Physical Vehicle/Path/Enabled ==
  VehFdbk : Inport
  Bus Selector : BusSelector  OutputSignals=VehFdbk.BdyFrm.Cg.Acc.ax,VehFdbk.BdyFrm.Cg.Acc.ay
  Constant5 : Constant
  Constant6 : Constant  Value=0
  Hypot : Math  Operator=hypot
  Saturation : Saturate  UpperLimit=1  LowerLimit=0  ZeroCross=off
  Simulation 3D Actor : sim3dlib/Simulation 3D Actor  ActorName=GamePhysVehPath  ParentName=Scene Origin  Operation=Create at setup  InitScriptText=|  SampleTime=Ts*5  Translation=[0 0 0]  Rotation=[0 0 0]  Scale=[1 1 1]  InputsText=PathMarker.Color  aMode=5  ActorTag=GamePhysVehPath  ActorType=Sim3dActor  ID=C
      | path1 = sim3d.graphics.PathMarker("ActorName", "PathMarker", ControlActorName="SimulinkVehicle2");
      | path1.MarkersSize = ones(1,3)*0.25;
      | path1.Color = [0 0 1];
      | World.add(path1,Actor);
  Sum1 : Sum  Inputs=|++
  Terminator4 : Terminator
  Unary Minus : UnaryMinus
  Vector Concatenate : Concatenate  NumInputs=3  Mode=Multidimensional array  ConcatenateDimension=2
  wires:
  Hypot/1 -> Saturation/1
  Saturation/1 -> Unary Minus/1, Vector Concatenate/1
  Constant5/1 -> Sum1/2
  Simulation 3D Actor/1 -> Terminator4/1
  Sum1/1 -> Vector Concatenate/3
  Unary Minus/1 -> Sum1/1
  Constant6/1 -> Vector Concatenate/2
  VehFdbk/1 -> Bus Selector/1
  Bus Selector/2 -> Hypot/2  "<ay>"
  Bus Selector/1 -> Hypot/1  "<ax>"
  Vector Concatenate/1 -> Simulation 3D Actor/1

== system manualInputSim/3D Visualization/Enabled/3D Visualization/Simulation 3D Vehicle/Annotations/Disabled ==
